simulink model "sim_circ_traj_tracking"  (R2024b)
settings: Solver=FixedStepAuto  StartTime=0.0  StopTime=total_time  RelTol=1e-3
values from neighbouring files (symbols this model uses):
  control_par = [k1, k2,b]    [init_circ_path_plannig.m]
  controller_index = 3    [init_circ_path_plannig.m]
  d = d_nominal    (= 0.165)    [init_circ_path_plannig.m]
  D = diag([0.001, 0.001, 0.001, 0.0175/6, 0.0175/6, 0.0175/6*T_s, 0.0175/6*T_s].^2)    [init_circ_path_plannig.m]
  d_actual = d_nominal    (= 0.165)    [init_circ_path_plannig.m]
  omega_M = 10    [init_circ_path_plannig.m]
  P_INIT_EKF = diag([0.001, 0.001, 0.001, 0.0175/6, 0.0175/6, 0.0175/6*T_s, 0.0175/6*T_s].^2)    [init_circ_path_plannig.m]
  prob_gps_loss = 0.9    [init_circ_path_plannig.m]
  qi = [1.45;-0.3;0]    [init_circ_path_plannig.m]
  r = r_nominal    (= 0.03)    [init_circ_path_plannig.m]
  R_2 = diag([ENCODER_QUANTIZATION/6,ENCODER_QUANTIZATION/6].^2)    [init_circ_path_plannig.m]
  R_5 = diag(([0.001, 0.001, 0.001, ENCODER_QUANTIZATION/6,ENCODER_QUANTIZATION/6]).^2)    [init_circ_path_plannig.m]
  r_actual = r_nominal    (= 0.03)    [init_circ_path_plannig.m]
  T_s = 0.04    [init_circ_path_plannig.m]
  Ts = 0.04    [init_circ_path_plannig.m]
undefined symbols (not defined in the file or in its folder): X, Y
libraries: robotlib x4, simulink x2, sharedtransform x1, dspsigops x1
settings Model: Creator=riccardo01  LastModifiedBy=defendenri
settings OptimizationCC: DefaultParameterBehavior=Inlined  EnhancedBackFolding=on  PassReuseOutputArgsAs=Individual arguments  ZeroExternalMemoryAtStartup=off  ZeroInternalMemoryAtStartup=off  MaxStackSize=64  OptimizeBlockOrder=speed  DifferentSizesBufferReuse=on  OptimizationCustomize=off  EfficientTunableParamExpr=on
settings DebuggingCC: ParameterTunabilityLossMsg=error
settings HardwareCC: ProdBitPerPointer=32  ProdBitPerSizeT=32  ProdBitPerPtrDiffT=32  ProdLargestAtomicFloat=None  ProdIntDivRoundTo=Undefined  ProdEndianess=Unspecified  ProdWordSize=32  ProdHWDeviceType=Generic->Unspecified (assume 32-bit Generic)
settings SFSimCC: MATLABDynamicMemAlloc=off
settings RTWCC: Description=Embedded Coder  SystemTargetFile=ert.tlc  HardwareBoard=Robot Operating System (ROS)  TLCOptions="-aInlineSetEventsForThisBaseRateFcn=TLC_FALSE -aSuppressMultiTaskScheduler=TLC_FALSE  -aRateBasedStepFcn=0"  TemplateMakefile=ert_default_tmf  Toolchain=Catkin  TargetLang=C++
settings CodeAppCC: ForceParamTrailComments=on  IgnoreCustomStorageClasses=off  OperatorAnnotations=on  SimulinkDataObjDesc=on  SFDataObjDesc=on  InsertBlockDesc=on

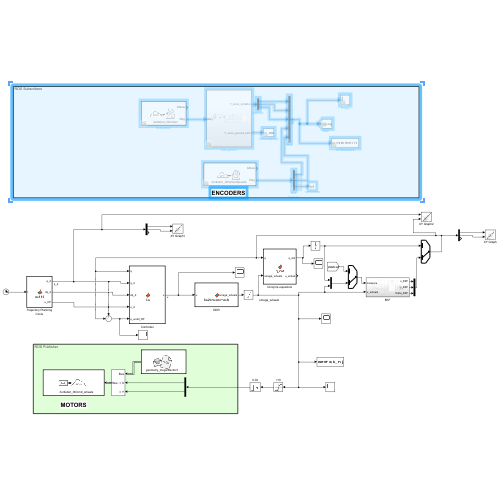
[thumbnail: Simulink's stored preview of the top-level diagram]
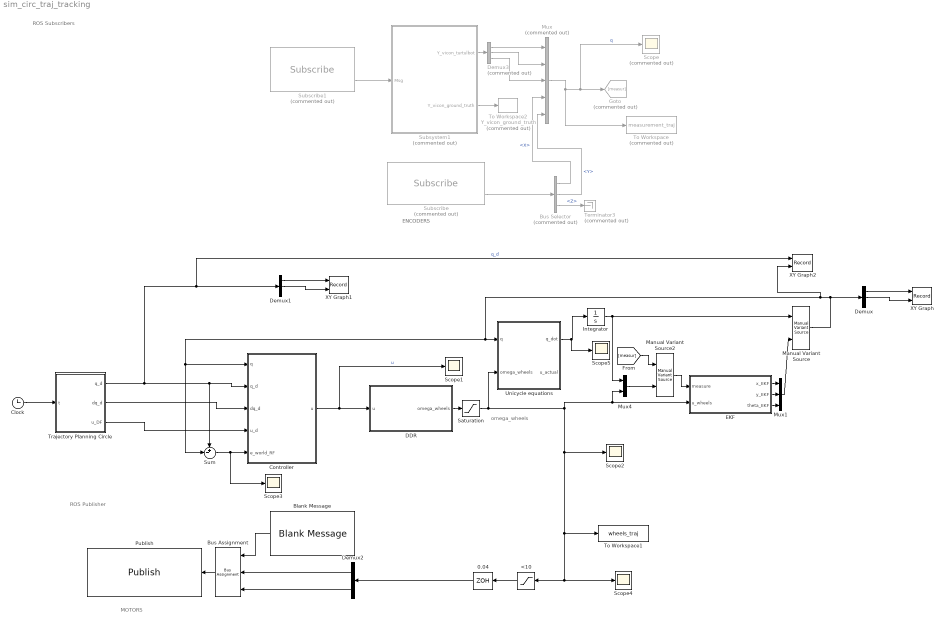
== system sim_circ_traj_tracking ==
  note: MOTORS
  note: ROS Publisher
  note: ROS Subscribers
  note: omega_wheels
  note: ENCODERS
  0.04 : ZeroOrderHold  SampleTime=Ts
  <10 : Saturate  UpperLimit=10  LowerLimit=-10
  Blank Message : robotlib/Blank Message  messageClass=Message  entityType=geometry_msgs/Vector3  messageType=geometry_msgs/Vector3  SampleTime=Ts  legacyBusStruct=off
      settings: LibrarySourceBlock=roslib/ROS/Blank Message
  Bus Assignment : BusAssignment  AssignedSignals=X,Y
  Bus Selector : BusSelector  Commented=on  OutputSignals=X,Y,Z
  Clock : Clock
      settings: Decimation=1/Ts
  Controller : MATLAB Function  TreatAsAtomicUnit=on
  DDR : MATLAB Function  TreatAsAtomicUnit=on
  Demux : Demux  Outputs=3
  Demux1 : Demux  Outputs=3
  Demux2 : Demux  Outputs=2
  Demux3 : Demux  Commented=on  Outputs=3
  EKF : Subsystem
  Goto : Goto  Commented=on  GotoTag=measur
  Integrator : Integrator  InitialCondition=qi
  Manual Variant Source : simulink/Signal Routing/Manual Variant Source  NumChoices=2  LabelModeActiveChoice=V_2
  Manual Variant Source2 : simulink/Signal Routing/Manual Variant Source  NumChoices=2  LabelModeActiveChoice=V_2
  Mux : Mux  Commented=on  Inputs=5
  Mux1 : Mux  Inputs=3
  Mux4 : Mux  Inputs=2
  Publish : robotlib/Publish  topicSource=Specify your own  topic=/turtlebot_06/cmd_wheels  messageType=geometry_msgs/Vector3  legacyBusStruct=off  messageQueueLength=1
      settings: LibrarySourceBlock=roslib/ROS/Publish
  Saturation : Saturate  UpperLimit=omega_M  LowerLimit=-omega_M
  Scope : Scope  Commented=on
  Scope{1..5} (5 alike) : Scope
  Subscribe : robotlib/Subscribe  Commented=on  topicSource=Specify your own  topic=/turtlebot_06/wheelSpeeds  messageType=geometry_msgs/Vector3  SampleTime=T_s  legacyBusStruct=off  messageQueueLength=1
      settings: LibrarySourceBlock=roslib/ROS/Subscribe
  Subscribe1 : robotlib/Subscribe  Commented=on  topicSource=Specify your own  topic=/turtlebot_06/odom  messageType=nav_msgs/Odometry  SampleTime=T_s  legacyBusStruct=off  messageQueueLength=1
      settings: LibrarySourceBlock=roslib/ROS/Subscribe
  Subsystem1 : Subsystem  Commented=on
  Sum : Sum  Inputs=+-|
  Terminator3 : Terminator  Commented=on
  To Workspace : ToWorkspace  Commented=on  VariableName=measurement_traj  SaveFormat=Timeseries  SampleTime=-1
  To Workspace1 : ToWorkspace  VariableName=wheels_traj  SaveFormat=Timeseries  SampleTime=-1
  To Workspace2 : ToWorkspace  Commented=on  VariableName=Y_vicon_ground_truth  SaveFormat=Timeseries  SampleTime=T_s
  Trajectory Planning Circle : MATLAB Function  TreatAsAtomicUnit=on
  Unicycle equations : MATLAB Function  TreatAsAtomicUnit=on
  XY Graph : Record  FileSettingsInternal="{\"entries\":[{\"content\":{\"excelSettings\":{\"content\":{},\"type\":\"Streamout.ExcelSettings\"}},\"type\":\"Streamout.FileSettingStorage\",\"uuid\":\"\"}],\"packageUris\":[\"http:\\/\\/schema.mathworks.com\\/mf0\\/streamout_blocks\\/R2020a\"],\"version\":\"1.0\"}"  Layout=[1 1]  SignalsInternal="{\"entries\":[{\"content\":{\"signals\":[{\"content\":{\"blockPath\":[],\"dimensions\":[1],\"domain\":\"\",\"lineColor\":\"#a2142f\",\"plots\":[ 1 ],\"port\":1,\"sid\":[\"\"],\"signalID\":1,\"signalName\":\"Demux:1\"},\"type\":\"RecordBlkView.Signal\",\"uuid\":\"\"},{\"content\":{\"blockPath\":[],\"dimensions\":[1],\"domain\":\"\",\"lineColor\":\"#139fff\",\"plots\":[ 1 ],\"port\":2,\"sid\":[\"\"],\"signalID\":2,\"signalName\":\"Demux:2\"},\"type\":\"RecordBlkView.Signal\",\"uuid\":\"\"}]},\"type\":\"RecordBlkView.InputSignals\",\"uuid\":\"\"}],\"packageUris\":[\"http:\\/\\/schema.mathworks.com\\/mf0\\/streamout_blocks\\/R2020a\"],\"version\":\"1.0\"}"  VisualizationBindings="{\"xyplotplugin\":{\"info\":[{\"series\":[{\"bindingParametersList\":[{\"parameter\":\"X-Axis\",\"signalID\":1,\"signalName\":\"Demux:1\"},{\"parameter\":\"Y-Axis\",\"signalID\":2,\"signalName\":\"Demux:2\"}],\"seriesID\":0}],\"subplotID\":1}]}}"  CompatibilityTag=XY
  XY Graph1 : Record  FileSettingsInternal="{\"entries\":[{\"content\":{\"excelSettings\":{\"content\":{},\"type\":\"Streamout.ExcelSettings\"}},\"type\":\"Streamout.FileSettingStorage\",\"uuid\":\"\"}],\"packageUris\":[\"http:\\/\\/schema.mathworks.com\\/mf0\\/streamout_blocks\\/R2020a\"],\"version\":\"1.0\"}"  Layout=[1 1]  SignalsInternal="{\"entries\":[{\"content\":{\"signals\":[{\"content\":{\"blockPath\":[],\"dimensions\":[1,1],\"domain\":\"\",\"lineColor\":\"#77ac30\",\"lineWidth\":2,\"plots\":[ 1 ],\"port\":1,\"sid\":[\"\"],\"signalID\":1,\"signalName\":\"Demux1:1\"},\"type\":\"RecordBlkView.Signal\",\"uuid\":\"\"},{\"content\":{\"blockPath\":[],\"dimensions\":[1,1],\"domain\":\"\",\"lineColor\":\"#4dbeee\",\"lineWidth\":2,\"plots\":[ 1 ],\"port\":2,\"sid\":[\"\"],\"signalID\":2,\"signalName\":\"Demux1:2\"},\"type\":\"RecordBlkView.Signal\",\"uuid\":\"\"}]},\"type\":\"RecordBlkView.InputSignals\",\"uuid\":\"\"}],\"packageUris\":[\"http:\\/\\/schema.mathworks.com\\/mf0\\/streamout_blocks\\/R2020a\"],\"version\":\"1.0\"}"  VisualizationBindings="{\"xyplotplugin\":{\"info\":[{\"series\":[{\"bindingParametersList\":[{\"parameter\":\"X-Axis\",\"signalID\":1,\"signalName\":\"Demux1:1\"},{\"parameter\":\"Y-Axis\",\"signalID\":2,\"signalName\":\"Demux1:2\"}],\"seriesID\":0}],\"subplotID\":1}]}}"  CompatibilityTag=XY
  XY Graph2 : Record  FileSettingsInternal="{\"entries\":[{\"content\":{\"excelSettings\":{\"content\":{},\"type\":\"Streamout.ExcelSettings\"}},\"type\":\"Streamout.FileSettingStorage\",\"uuid\":\"\"}],\"packageUris\":[\"http:\\/\\/schema.mathworks.com\\/mf0\\/streamout_blocks\\/R2020a\"],\"version\":\"1.0\"}"  Layout=[1 1]  SignalsInternal="{\"entries\":[{\"content\":{\"signals\":[{\"content\":{\"blockPath\":[],\"dimensions\":[3,1],\"domain\":\"\",\"hasChildren\":true,\"lineColor\":\"#139fff\",\"lineWidth\":2,\"port\":1,\"sid\":[\"\"],\"signalID\":1,\"signalName\":\"q_d\"},\"type\":\"RecordBlkView.Signal\",\"uuid\":\"\"},{\"content\":{\"blockPath\":[],\"channel\":[1,1],\"dimensions\":[3,1],\"domain\":\"\",\"lineColor\":\"#b746ff\",\"lineWidth\":2,\"parentID\":1,\"plots\":[ 1 ],\"port\":1,\"sid\":[\"\"],\"signalID\":2,\"signalName\":\"q_d\"},\"type\":\"RecordBlkView.Signal\",\"uuid\":\"\"},{\"content\":{\"blockPath\":[],\"dimensions\":[3],\"domain\":\"\",\"hasChildren\":true,\"lineColor\":\"#b746ff\",\"lineWidth\":2,\"port\":2,\"sid\":[\"\"],\"signalID\":3},\"type\":\"RecordBlkView.Signal\",\"uuid\":\"\"},{\"content\":{\"blockPath\":[],\"channel\":[1],\"dimensions\":[3],\"domain\":\"\",\"lineColor\":\"#ff13a6\",\"lineWidth\":2,\"parentID\":3,\"plots\":[ 1 ],\"port\":2,\"sid\":[\"\"],\"signalID\":4},\"type\":\"RecordBlkView.Signal\",\"uuid\":\"\"},{\"content\":{\"blockPath\":[],\"channel\":[2,1],\"dimensions\":[3,1],\"domain\":\"\",\"lineColor\":\"#0072bd\",\"lineWidth\":2,\"parentID\":1,\"plots\":[ 1 ],\"port\":1,\"sid\":[\"\"],\"signalID\":5,\"signalName\":\"q_d\"},\"type\":\"RecordBlkView.Signal\",\"uuid\":\"\"},{\"content\":{\"blockPath\":[],\"channel\":[3,1],\"dimensions\":[3,1],\"domain\":\"\",\"lineColor\":\"#d95319\",\"lineWidth\":2,\"parentID\":1,\"port\":1,\"sid\":[\"\"],\"signalID\":6,\"signalName\":\"q_d\"},\"type\":\"RecordBlkView.Signal\",\"uuid\":\"\"},{\"content\":{\"blockPath\":[],\"channel\":[2],\"dimensions\":[3],\"domain\":\"\",\"lineColor\":\"#edb120\",\"lineWidth\":2,\"parentID\":3,\"plots\":[ 1 ],\"port\":2,\"sid\":[\"\"],\"signalID\":7},\"type\":\"RecordBlkView.Signal\",\"uuid\":\"\"},{\"content\":{\"blockPath\":[],\"channel\":[3],\"dimensions\":[3],\"domain\":\"\",\"lineColor\":\"#7e2f8e\",\"lineWidth\":2,\"parentID\":3,\"port\":2,\"sid\":[\"\"],\"signalID\":8},\"type\":\"RecordBlkView.Signal\",\"uuid\":\"\"}]},\"type\":\"RecordBlkView.InputSignals\",\"uuid\":\"\"}],\"packageUris\":[\"http:\\/\\/schema.mathworks.com\\/mf0\\/streamout_blocks\\/R2020a\"],\"version\":\"1.0\"}"  VisualizationBindings="{\"xyplotplugin\":{\"info\":[{\"series\":[{\"bindingParametersList\":[{\"parameter\":\"X-Axis\",\"signalID\":4,\"signalName\":\"XY Graph2:2(1)\"},{\"parameter\":\"Y-Axis\",\"signalID\":7,\"signalName\":\"XY Graph2:2(2)\"}],\"seriesID\":0},{\"bindingParametersList\":[{\"parameter\":\"X-Axis\",\"signalID\":2,\"signalName\":\"q_d(1,1)\"},{\"parameter\":\"Y-Axis\",\"signalID\":5,\"signalName\":\"q_d(2,1)\"}],\"seriesID\":1}],\"subplotID\":1}]}}"  CompatibilityTag=XY
  wires:
  0.04/1 -> Demux2/1
  Blank Message/1 -> Bus Assignment/1
  <10/1 -> 0.04/1
  Demux2/2 -> Bus Assignment/3
  Bus Assignment/1 -> Publish/1
  Demux2/1 -> Bus Assignment/2
  Saturation/1 -> Unicycle equations/2(omega_wheels), Scope2/1, To Workspace1/1, <10/1, Scope4/1, EKF/2(u_wheels), Mux4/2
  EKF/2(y_EKF) -> Mux1/2
  EKF/1(x_EKF) -> Mux1/1
  EKF/3(theta_EKF) -> Mux1/3
  Sum/1 -> Scope3/1, Controller/5(e_world_RF)
  Controller/1(u) -> Scope1/1, DDR/1(u)  "u"
  Unicycle equations/1(q_dot) -> Scope5/1, Integrator/1
  Demux/1 -> XY Graph/1
  Demux/2 -> XY Graph/2
  Demux1/1 -> XY Graph1/1
  Demux1/2 -> XY Graph1/2
  DDR/1(omega_wheels) -> Saturation/1
  Manual Variant Source/1 -> XY Graph2/2, Controller/1(q), Sum/2, Unicycle equations/1(q), Demux/1
  Integrator/1 -> Manual Variant Source/1, Mux4/1
  Mux1/1 -> Manual Variant Source/2
  Clock/1 -> Trajectory Planning Circle/1(t)
  Trajectory Planning Circle/3(u_DF) -> Controller/4(u_d)
  Trajectory Planning Circle/2(dq_d) -> Controller/3(dq_d)
  Trajectory Planning Circle/1(q_d) -> Demux1/1, XY Graph2/1, Controller/2(q_d), Sum/1  "q_d"
  Mux4/1 -> Manual Variant Source2/2
  [measur] -> Manual Variant Source2/1
  Manual Variant Source2/1 -> EKF/1(measure)
  Subscribe1/2 -> Subsystem1/1(Msg)
  Subsystem1/1(Y_vicon_turtulbot) -> Demux3/1
  Bus Selector/3 -> Terminator3/1  "<Z>"
  Bus Selector/1 -> Mux/4  "<X>"
  Bus Selector/2 -> Mux/5  "<Y>"
  Subscribe/2 -> Bus Selector/1
  Mux/1 -> To Workspace/1, Goto/1, Scope/1  "q"
  Demux3/1 -> Mux/1
  Demux3/2 -> Mux/2
  Demux3/3 -> Mux/3
  Subsystem1/2(Y_vicon_ground_truth) -> To Workspace2/1

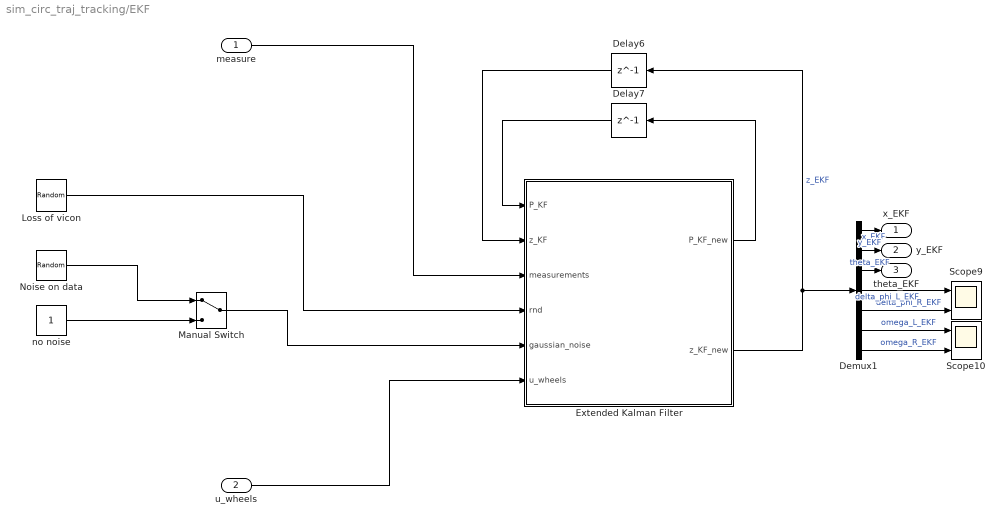
== system sim_circ_traj_tracking/EKF ==
  measure : Inport
  u_wheels : Inport  Port=2
  " Loss of vicon" : UniformRandomNumber  Minimum=0
  Delay6 : Delay  DelayLength=1  InitialCondition=[qi; 0; 0; 0; 0]
  Delay7 : Delay  DelayLength=1  InitialCondition=P_INIT_EKF
  Demux1 : Demux  Outputs=7
  Extended Kalman Filter : MATLAB Function  TreatAsAtomicUnit=on
  Manual Switch : ManualSwitch
  Noise on data : RandomNumber  Variance=0.0001
  Scope10 : Scope  NumInputPorts=2
  Scope9 : Scope  NumInputPorts=2
  no noise : Constant
  x_EKF : Outport
  y_EKF : Outport  Port=2
  theta_EKF : Outport  Port=3
  wires:
  Demux1/6 -> Scope10/1  "omega_L_EKF"
  Demux1/3 -> theta_EKF/1  "theta_EKF"
  Delay6/1 -> Extended Kalman Filter/2(z_KF)
  Delay7/1 -> Extended Kalman Filter/1(P_KF)
  Noise on data/1 -> Manual Switch/1
  Demux1/5 -> Scope9/2  "delta_phi_R_EKF"
  Demux1/7 -> Scope10/2  "omega_R_EKF"
  Extended Kalman Filter/1(P_KF_new) -> Delay7/1
  Manual Switch/1 -> Extended Kalman Filter/5(gaussian_noise)
  " Loss of vicon"/1 -> Extended Kalman Filter/4(rnd)
  Demux1/1 -> x_EKF/1  "x_EKF"
  Demux1/4 -> Scope9/1  "delta_phi_L_EKF"
  no noise/1 -> Manual Switch/2
  u_wheels/1 -> Extended Kalman Filter/6(u_wheels)
  Extended Kalman Filter/2(z_KF_new) -> Demux1/1, Delay6/1  "z_EKF"
  measure/1 -> Extended Kalman Filter/3(measurements)
  Demux1/2 -> y_EKF/1  "y_EKF"

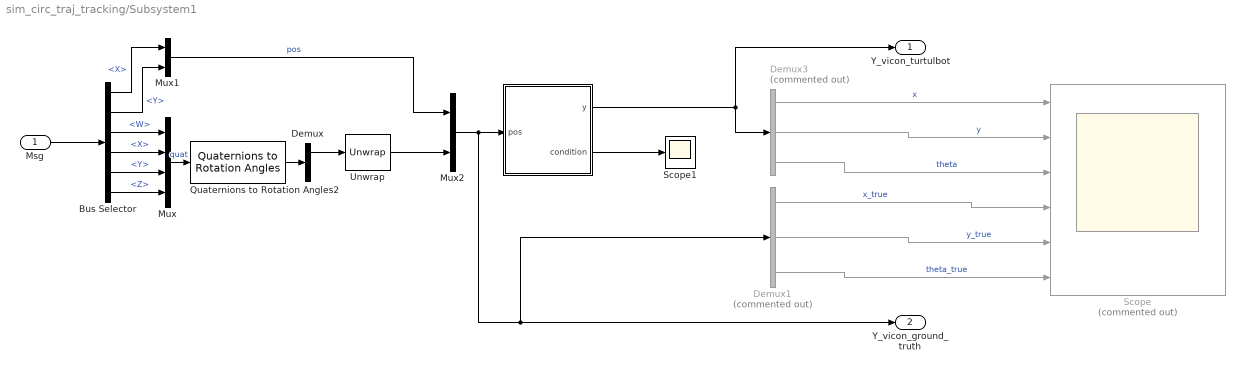
== system sim_circ_traj_tracking/Subsystem1 ==
  Msg : Inport
  " " : MATLAB Function  TreatAsAtomicUnit=on
  Bus Selector : BusSelector  OutputSignals=Pose.Pose.Position.X,Pose.Pose.Position.Y,Pose.Pose.Orientation.W,Pose.Pose.Orientation.X,Pose.Pose.Orientation.Y,Pose.Pose.Orientation.Z
  Demux : Demux  Outputs=3
  Demux1 : Demux  Commented=on  Outputs=3
  Demux3 : Demux  Commented=on  Outputs=3
  Mux : Mux
  Mux1 : Mux  Inputs=2
  Mux2 : Mux  Inputs=2
  Quaternions to Rotation Angles2 : sharedtransform/Quaternions to Rotation Angles  rotationOrder=ZYX  aMode=aMode
  Scope : Scope  Commented=on  NumInputPorts=6
  Scope1 : Scope
  Unwrap : dspsigops/Unwrap  tol=pi  InputProcessing=Columns as channels (frame based)  running=off
  Y_vicon_turtulbot : Outport
  Y_vicon_ground_truth : Outport  Port=2
  wires:
  Demux/1 -> Unwrap/1
  Quaternions to Rotation Angles2/1 -> Demux/1
  Mux1/1 -> Mux2/1  "pos"
  Unwrap/1 -> Mux2/2
  Demux1/1 -> Scope/4  "x_true"
  Demux3/2 -> Scope/2  "y"
  Demux3/3 -> Scope/3  "theta"
  " "/2(condition) -> Scope1/1
  Demux1/3 -> Scope/6  "theta_true"
  Bus Selector/5 -> Mux/3  "<Y>"
  Bus Selector/4 -> Mux/2  "<X>"
  Demux1/2 -> Scope/5  "y_true"
  " "/1(y) -> Demux3/1, Y_vicon_turtulbot/1
  Bus Selector/1 -> Mux1/1  "<X>"
  Bus Selector/6 -> Mux/4  "<Z>"
  Demux3/1 -> Scope/1  "x"
  Bus Selector/2 -> Mux1/2  "<Y>"
  Mux/1 -> Quaternions to Rotation Angles2/1  "quat"
  Bus Selector/3 -> Mux/1  "<W>"
  Mux2/1 -> " "/1(pos), Y_vicon_ground_truth/1, Demux1/1
  Msg/1 -> Bus Selector/1

== matlab function sim_circ_traj_tracking/Controller ==
  data: q input; q_d input; dq_d input; u_d input; u output; e_world_RF input; controller_index parameter; control_par parameter
function u  = fcn(q, q_d, dq_d, u_d, e_world_RF, controller_index, control_par)
% compute the error in the unicycle RF
M=[ cos(q(3)),  sin(q(3)),  0;
    -sin(q(3)), cos(q(3)),  0;
    0,               0,       1];
e=M*e_world_RF;

e(3)=wrapToPi(e(3));

if controller_index == 1
    % linear controller
    %control_par = [xi, a, 0];
    if u_d(1)<=10^-3 && u_d(1)>=-10^-3
        u_d(1)=10^-3;
    end
    
    k3 = 2*control_par(1)*control_par(2);
    k1 = k3;
    k2 = (control_par(2)^2 - u_d(2)^2)/u_d(1);
    u = [k1*e(1) + cos(e(3))*u_d(1); 
        k2*e(2)+k3*e(3) + u_d(2)];

    

elseif controller_index == 2
    % nonlinear controller
    %control_par = [xi, b, 0];
    %singularity avoidance
    if e(3)<=10^-3 && e(3)>=-10^-3
        e(3)=10^-3;
    end

    k2 = control_par(2);
    
    k1 = 2*control_par(1)*sqrt(u_d(1)*control_par(2) + u_d(2)^2);
    k3 = k1;

    u = [k1*e(1)+ cos(e(3))*u_d(1);
        k2*(u_d(1)*sin(e(3))/e(3))*e(2) + k3*e(3)+ u_d(2)];
    


elseif controller_index == 3
    % feedback linearization
    %control_par = [k1, k2,b];
    k1=control_par(1);
    k2=control_par(2);
    b=control_par(3);

    v=u_d(1);
    w=u_d(2);

    %evaluation b point
    Xb=q(1)+b*cos(q(3));
    Yb=q(2)+b*sin(q(3));

    %evaluation b point desired
    Xb_d=q_d(1)+b*cos(q_d(3));
    Yb_d=q_d(2)+b*sin(q_d(3));

    %evaluation derivatives b point desired
    dXb_d=dq_d(1)-b*sin(q_d(3))*dq_d(3);
    dYb_d=dq_d(2)+b*cos(q_d(3))*dq_d(3);

    %matrix b poit to point
    T_inv=[ cos(q(3)),      sin(q(3));
            -sin(q(3))/b,   cos(q(3))/b];

    %evaluation of controll law
    u = T_inv*[ dXb_d+k1*(Xb_d-Xb);
                dYb_d+k2*(Yb_d-Yb)];

    % u = [v*cos(q_d(3)-q(3)) + b*dq_d(3)*sin(q_d(3)-q(3));
    %     dq_d(3)*cos(q_d(3)-q(3)) + v*sin(q_d(3)-q(3))/b];
else
    u = u_d;
end

== matlab function sim_circ_traj_tracking/DDR ==
  data: u input; omega_wheels output; r parameter; d parameter; omega_M parameter
function omega_wheels = kin2omegawheels(u, r, d, omega_M)
omega_l = u(1)/r-d/(2*r)*u(2);
omega_r = u(1)/r+d/(2*r)*u(2);
if (abs(omega_l)>=omega_M)||(abs(omega_r)>=omega_M)%if atleast one of the weel is in saturation
    W_m=max([abs(omega_l),abs(omega_r)]);
  
    omega_l=(omega_l/W_m)*omega_M;
    omega_r=(omega_r/W_m)*omega_M;
end

omega_wheels = [omega_l;omega_r];
end

== matlab function sim_circ_traj_tracking/Unicycle equations ==
  data: q input; omega_wheels input; q_dot output; r_actual parameter; d_actual parameter; u_actual output
function [q_dot, u_actual] = q_dot(q, omega_wheels, r_actual, d_actual)
u_actual = [r_actual/2, r_actual/2;-r_actual/d_actual, r_actual/d_actual]*omega_wheels;
theta = q(3);
q_dot = [[cos(theta), 0];[sin(theta), 0];[0,1]]*u_actual;

== matlab function sim_circ_traj_tracking/Subsystem1/  ==
  data: y output; pos input; condition output
function [y, condition] = check(pos)

x1 = -2.9; y1 = -1.5;
x2 = -1.6; y2 = -1.1;
x3 = -1.5; y3 = -0.7;
x4 = -1.4; y4 = -0.3;
x5 = -0.6; y5 =  0.1;
x6 =  0.2; y6 =  1.5;
x7 =  1.0;
x8 =  1.1;
x9 =  2.9;

P_loss = 0.9;


if ((pos(1) >= x5) && (pos(1) <= x6)) && ((pos(2) >= y1) && (pos(2) <= y5))
    % add noise
    y = pos + 0.02*randn(3,1);
    condition = 1;
elseif ((pos(1) >= x7) && (pos(1) <= x9)) && ((pos(2) >= y1) && (pos(2) <= y6))
    % measurement loss
    if rand > P_loss
        y = pos;
    else
        y = 0*pos;
    end
    condition = 2;
else
    y = pos;
    condition = 0;
end

== matlab function sim_circ_traj_tracking/Trajectory Planning Circle ==
  data: t input; q_d output; dq_d output; u_DF output; T_trj parameter
function [q_d, dq_d, u_DF] = get_trj(t, T_trj)
    % circle
    center=[2,0];
    qi=[1.45,-0.3,0];
    delta_x=qi(1)-center(1);
    delta_y=qi(2)-center(2);
    r =sqrt((delta_x)^2+(delta_y)^2);%distance from initial point to center
    omega = 3*pi/T_trj;
    pi_0=atan2(delta_y,delta_x);

    theta_prime = omega*t+pi_0;
    q_d = [r*cos(theta_prime)+2; r*sin(theta_prime); theta_prime + pi/2];
    dq_d = [-omega*r*sin(theta_prime); omega*r*cos(theta_prime); omega];
    u_DF = [omega*r; omega];

== matlab function sim_circ_traj_tracking/EKF/Extended Kalman Filter ==
  data: P_KF input; P_KF_new output; z_KF input; measurements input; D parameter; R_2 parameter; R_5 parameter; Ts parameter; r parameter; d parameter; prob_gps_loss parameter; rnd input; gaussian_noise input; z_KF_new output; u_wheels input
function [P_KF_new, z_KF_new] = EKF_filtering(P_KF, z_KF, measurements, D, R_2, R_5 ,Ts, r, d, prob_gps_loss, rnd, gaussian_noise,u_wheels)


% z_KF = [x_EKF, y_EKF, theta_EKF, delta_phi_L_EKF, delta_phi_R_EKF, omega_L_EKF, omega_R_EKF]

v_k = r * (z_KF(6) + z_KF(7))/2;
w_k = r * (z_KF(7) - z_KF(6))/d;

theta_mean = z_KF(3) + (w_k * Ts)/2;

F_k = [1, 0, -Ts * v_k * sin(theta_mean), 0, 0, Ts * r * cos(theta_mean)/2 + (Ts)^2 * r * v_k * sin(theta_mean)/(2*d), Ts * r * cos(theta_mean)/2 - (Ts)^2 * r * v_k * sin(theta_mean)/(2*d);
       0, 1,  Ts * v_k * cos(theta_mean), 0, 0, Ts * r * sin(theta_mean)/2 + (Ts)^2 * r * v_k * cos(theta_mean)/(2*d), Ts * r * sin(theta_mean)/2 - (Ts)^2 * r * v_k * cos(theta_mean)/(2*d);
       0, 0, 1, 0, 0, (-Ts*r)/d, (Ts*r)/d;
       0, 0, 0, 0, 0, Ts, 0;
       0, 0, 0, 0, 0, 0, Ts;
       0, 0, 0, 0, 0, 0, 0;
       0, 0, 0, 0, 0, 0, 0];

%% Prediction part

z_pred = [z_KF(1)+(Ts*r*(z_KF(6)+z_KF(7))/2)*cos(theta_mean + (Ts*r*(z_KF(6)+z_KF(7)))/(2*d));
          z_KF(2)+(Ts*r*(z_KF(6)+z_KF(7))/2)*sin(theta_mean + (Ts*r*(z_KF(7)-z_KF(6)))/(2*d));
          theta_mean + (Ts*r*(z_KF(7)-z_KF(6))/(2*d));
          Ts*z_KF(6);
          Ts*z_KF(7);
          u_wheels(1);
          u_wheels(2)];

P_pred = F_k * P_KF * F_k' + D;


%% Update

    % GPS(x,y,yaw) + Encoders(omegaL,omegaR)
    y_measurement = [measurements(1)+gaussian_noise;measurements(2)+gaussian_noise;measurements(3)+gaussian_noise; measurements(4); measurements(5)];
    
    H = [1, 0, 0, 0, 0, 0, 0;
         0, 1, 0, 0, 0, 0, 0;
         0, 0, 1, 0, 0, 0, 0;
         0, 0, 0, 0, 0, 1, 0;
         0, 0, 0, 0, 0, 0, 1];

    e = y_measurement - H * z_pred;
    K = P_pred * H' /(H * P_pred * H' + R_5);

    z_KF_new = z_pred + K * e;
    P_KF_new = P_pred - K * H * P_pred;

end
